simulink model "inverter"  (R2019b)
settings: Solver=VariableStepAuto  StartTime=0.0  StopTime=0.06  RelTol=1e-3
libraries: powerlib x17, powerlib_meascontrol x8
settings Model: Creator=96547  LastModifiedBy=96547

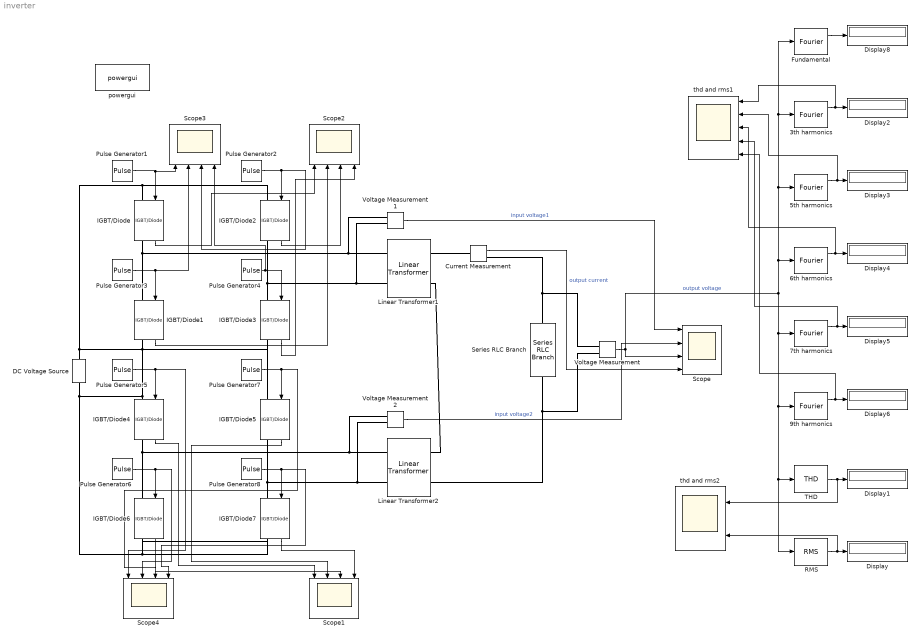
== system inverter ==
  3th harmonics : powerlib_meascontrol/Measurements/Fourier  Freq=50  n=3  InInit=[0, 0]  Ts=0
      settings: SourceProductName=Simscape Electrical
  5th harmonics : powerlib_meascontrol/Measurements/Fourier  Freq=50  n=5  InInit=[0, 0]  Ts=0
      settings: SourceProductName=Simscape Electrical
  6th harmonics : powerlib_meascontrol/Measurements/Fourier  Freq=50  n=6  InInit=[0, 0]  Ts=0
      settings: SourceProductName=Simscape Electrical
  7th harmonics : powerlib_meascontrol/Measurements/Fourier  Freq=50  n=7  InInit=[0, 0]  Ts=0
      settings: SourceProductName=Simscape Electrical
  9th harmonics : powerlib_meascontrol/Measurements/Fourier  Freq=50  n=9  InInit=[0, 0]  Ts=0
      settings: SourceProductName=Simscape Electrical
  Current Measurement : powerlib/Measurements/Current Measurement  PhasorSimulation=off  OutputType=Complex  PSBequivalent=0
      settings: SourceProductName=Simscape Electrical
  DC Voltage Source : powerlib/Electrical Sources/DC Voltage Source  Amplitude=400  Measurements=None
      settings: SourceProductName=Simscape Electrical
  Display{,1..6,8} (8 alike) : Display
  Fundamental : powerlib_meascontrol/Measurements/Fourier  Freq=50  n=1  InInit=[0, 0]  Ts=0
      settings: SourceProductName=Simscape Electrical
  IGBT/Diode{,1..7} (8 alike) : powerlib/Power Electronics/IGBT//Diode  Ron=0  Rs=1e5  Cs=inf  Measurements=on
      settings: SourceProductName=Simscape Electrical
  Linear Transformer1 : powerlib/Elements/Linear Transformer  UNITS=pu  NominalPower=[ 250e6 50 ]  winding1="[ 315e3  0  0 ]"  winding2="[ 315e3  0  0 ]"  ThreeWindings=off  winding3=[ 315e3 0.002 0.08 ]  RmLm=[ 500 500 ]  Measurements=None  DataType=off
      settings: SourceProductName=Simscape Electrical
  Linear Transformer2 : powerlib/Elements/Linear Transformer  UNITS=pu  NominalPower=[ 250e6 50 ]  winding1="[ 315e3  0  0 ]"  winding2="[ 315e3  0  0 ]"  ThreeWindings=off  winding3=[ 315e3 0.002 0.08 ]  RmLm=[ 500 500 ]  Measurements=None  DataType=off
      settings: SourceProductName=Simscape Electrical
  Pulse Generator1 : DiscretePulseGenerator  PulseType=Time based  Period=0.02  PulseWidth=50
  Pulse Generator2 : DiscretePulseGenerator  PulseType=Time based  Period=0.02  PulseWidth=50  PhaseDelay=0.02*(1/6)
  Pulse Generator3 : DiscretePulseGenerator  PulseType=Time based  Period=0.02  PulseWidth=50  PhaseDelay=0.01
  Pulse Generator4 : DiscretePulseGenerator  PulseType=Time based  Period=0.02  PulseWidth=50  PhaseDelay=0.01+0.02*(1/6)
  Pulse Generator5 : DiscretePulseGenerator  PulseType=Time based  Period=0.02  PulseWidth=50  PhaseDelay=60/360*0.02
  Pulse Generator6 : DiscretePulseGenerator  PulseType=Time based  Period=0.02  PulseWidth=50  PhaseDelay=60/360*0.02+0.01
  Pulse Generator7 : DiscretePulseGenerator  PulseType=Time based  Period=0.02  PulseWidth=50  PhaseDelay=60/360*0.02+0.02/6
  Pulse Generator8 : DiscretePulseGenerator  PulseType=Time based  Period=0.02  PulseWidth=50  PhaseDelay=60/360*0.02+0.02/6+0.01
  RMS : powerlib_meascontrol/Measurements/RMS  TrueRMS=on  Freq=60  RMSInit=120  Ts=0
      settings: SourceProductName=Simscape Electrical
  Scope{,1..4} (5 alike) : Scope  NumInputPorts=4
  Series RLC Branch : powerlib/Elements/Series RLC Branch  LConnTagsString=__new0  RConnTagsString=__new0  BranchType=R  Resistance=8  Inductance=1e-3  SetiL0=off  InitialCurrent=0  Capacitance=1e-6  Setx0=off  InitialVoltage=0  Measurements=None
      settings: SourceProductName=Simscape Electrical
  THD : powerlib_meascontrol/Measurements/THD  Freq=50  Ts=0
      settings: SourceProductName=Simscape Electrical
  Voltage Measurement : powerlib/Measurements/Voltage Measurement  PhasorSimulation=off  OutputType=Complex  PSBequivalent=0
      settings: SourceProductName=Simscape Electrical
  Voltage Measurement1 : powerlib/Measurements/Voltage Measurement  PhasorSimulation=off  OutputType=Complex  PSBequivalent=0
      settings: SourceProductName=Simscape Electrical
  Voltage Measurement2 : powerlib/Measurements/Voltage Measurement  PhasorSimulation=off  OutputType=Complex  PSBequivalent=0
      settings: SourceProductName=Simscape Electrical
  powergui : powerlib/powergui  Priority=1  SimulationMode=Continuous  SampleTime=50e-6  frequency=60  Iterations=50  frequencyindice=0  Pbase=100e6  ErrMax=1e-4  UnitsV=kV  UnitsW=MW  buscounter=0  FunctionMessages=off  echomessages=off  EnableUseOfTLC=off  CurrentSourceSwitches=off  DisableSnubberDevices=off  DisableRonSwitches=off  DisableVfSwitches=off  DisplayEquations=off  AutomaticDiscreteSolvers=off  SolverType=Tustin/Backward Euler (TBE)  Interpol=off  ExternalGateDelay=off  methode=off  Ts=100  x0status=blocks  SPID=on  SwTol=0  HookPort=off  NonlinearTolerance=1e-4  nMaxIteration=100  ContinueOnMaxIteration=off  RestoreLinks=warning  ResistiveCurrentMeasurement=off  Frange=[0:2:500]  Ylog=off  Xlog=on  ShowGrid=off  save=off  variable=ZData  structure=0  ZoomFFT=off  StartTime=0.0  cycles=1  DisplayStyle=1  fundamental=60  FreqAxis=off  MaxFrequency=1000  frequencyindicesteady=1  RmsSteady=1  display=off
      settings: SourceProductName=Simscape Electrical
  thd and rms1 : Scope  NumInputPorts=5
  thd and rms2 : Scope  NumInputPorts=2
  wires:
  Pulse Generator1/1 -> Scope3/1, IGBT/Diode/1
  Pulse Generator2/1 -> Scope3/3, IGBT/Diode2/1
  Pulse Generator3/1 -> Scope3/2, IGBT/Diode1/1
  Pulse Generator4/1 -> IGBT/Diode3/1, Scope3/4
  Pulse Generator7/1 -> Scope4/3, IGBT/Diode5/1
  Pulse Generator6/1 -> Scope4/2, IGBT/Diode6/1
  Pulse Generator5/1 -> Scope4/1, IGBT/Diode4/1
  Pulse Generator8/1 -> IGBT/Diode7/1, Scope4/4
  Voltage Measurement1/1 -> Scope/1  "input voltage1"
  Voltage Measurement2/1 -> Scope/2  "input voltage2"
  IGBT/Diode/1 -> Scope2/1
  Fundamental/1 -> Display8/1
  Voltage Measurement/1 -> RMS/1, THD/1, 9th harmonics/1, 7th harmonics/1, Fundamental/1, 3th harmonics/1, 5th harmonics/1, 6th harmonics/1, Scope/3  "output voltage"
  5th harmonics/1 -> thd and rms1/2, Display3/1
  THD/1 -> thd and rms2/1, Display1/1
  9th harmonics/1 -> Display6/1, thd and rms1/5
  6th harmonics/1 -> Display4/1, thd and rms1/3
  7th harmonics/1 -> thd and rms1/4, Display5/1
  3th harmonics/1 -> thd and rms1/1, Display2/1
  RMS/1 -> thd and rms2/2, Display/1
  IGBT/Diode2/1 -> Scope2/3
  IGBT/Diode1/1 -> Scope2/2
  IGBT/Diode3/1 -> Scope2/4
  IGBT/Diode4/1 -> Scope1/1
  IGBT/Diode5/1 -> Scope1/2
  IGBT/Diode6/1 -> Scope1/3
  IGBT/Diode7/1 -> Scope1/4
  Current Measurement/1 -> Scope/4  "output current"
  connections:
  IGBT/Diode/RConn1 -- Voltage Measurement1/LConn1 -- Linear Transformer1/LConn1 -- IGBT/Diode1/LConn1
  IGBT/Diode2/RConn1 -- Linear Transformer1/LConn2 -- Voltage Measurement1/LConn2 -- IGBT/Diode3/LConn1
  IGBT/Diode4/RConn1 -- Voltage Measurement2/LConn1 -- Linear Transformer2/LConn1 -- IGBT/Diode6/LConn1
  IGBT/Diode5/RConn1 -- Linear Transformer2/LConn2 -- Voltage Measurement2/LConn2 -- IGBT/Diode7/LConn1
  IGBT/Diode4/LConn1 -- IGBT/Diode5/LConn1 -- IGBT/Diode2/LConn1 -- IGBT/Diode/LConn1 -- DC Voltage Source/RConn1
  IGBT/Diode6/RConn1 -- IGBT/Diode3/RConn1 -- IGBT/Diode1/RConn1 -- DC Voltage Source/LConn1 -- IGBT/Diode7/RConn1
  Linear Transformer2/RConn1 -- Linear Transformer1/RConn2
  Linear Transformer2/RConn2 -- Series RLC Branch/RConn1 -- Voltage Measurement/LConn2
  Current Measurement/LConn1 -- Linear Transformer1/RConn1
  Current Measurement/RConn1 -- Voltage Measurement/LConn1 -- Series RLC Branch/LConn1
